simulink model "P3"  (R2023b)
settings: Solver=VariableStepAuto  StartTime=0.0  StopTime=10.0  MaxStep=0.001  RelTol=1e-3
values from neighbouring files (symbols this model uses):
  b1 = 1000    [P3parametros.m]    (also in ST.m)
  k1 = 16182    [P3parametros.m]    (also in ST.m)
  k2 = 19000    [P3parametros.m]    (also in ST.m)
  m1 = 290    [P3parametros.m]    (also in ST.m)
  m2 = 59    [P3parametros.m]    (also in ST.m)
settings Model: Creator=aquet  LastModifiedBy=aquet

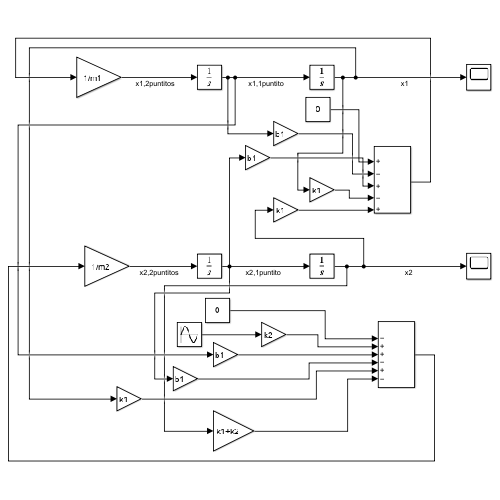
[thumbnail: Simulink's stored preview of the top-level diagram]
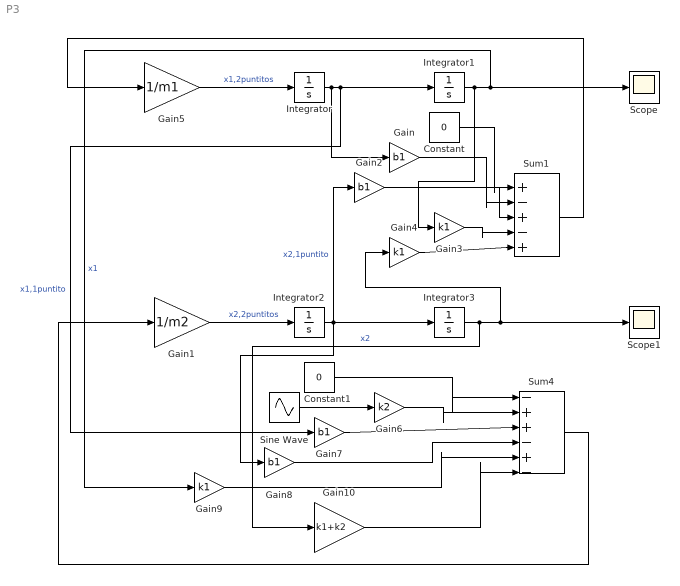
== system P3 ==
  Constant : Constant  Value=0
  Constant1 : Constant  Value=0
  Gain{,2,7..8} (4 alike) : Gain  Gain=b1
  Gain1 : Gain  Gain=1/m2
  Gain10 : Gain  Gain=k1+k2
  Gain3 : Gain  Gain=k1
  Gain4 : Gain  Gain=k1
  Gain5 : Gain  Gain=1/m1
  Gain6 : Gain  Gain=k2
  Gain9 : Gain  Gain=k1
  Integrator{,1..3} (4 alike) : Integrator
  Scope : Scope
  Scope1 : Scope
  Sine Wave : Sin  Amplitude=0.05  Frequency=0.5*pi  SampleTime=0
  Sum1 : Sum  Inputs=|+-+-+
  Sum4 : Sum  Inputs=|-++-+-
  wires:
  Gain5/1 -> Integrator/1  "x1,2puntitos"
  Integrator/1 -> Gain/1, Gain7/1, Integrator1/1  "x1,1puntito"
  Integrator1/1 -> Gain3/1, Gain9/1, Scope/1  "x1"
  Integrator2/1 -> Integrator3/1, Gain2/1, Gain8/1  "x2,1puntito"
  Gain1/1 -> Integrator2/1  "x2,2puntitos"
  Integrator3/1 -> Gain10/1, Gain4/1, Scope1/1  "x2"
  Constant1/1 -> Sum4/1
  Gain6/1 -> Sum4/2
  Gain7/1 -> Sum4/3
  Gain8/1 -> Sum4/4
  Gain9/1 -> Sum4/5
  Gain10/1 -> Sum4/6
  Sum4/1 -> Gain1/1
  Sine Wave/1 -> Gain6/1
  Constant/1 -> Sum1/1
  Gain/1 -> Sum1/2
  Gain2/1 -> Sum1/3
  Gain3/1 -> Sum1/4
  Gain4/1 -> Sum1/5
  Sum1/1 -> Gain5/1
